simulink model "rect_design"  (R2016a)
settings: Solver=ode4  StartTime=0.0  StopTime=0.5  FixedStep=1e-5  RelTol=1e-3
undefined symbols (not defined in the file or in its folder): Lload
libraries: powerlib x12, powerlib_meascontrol x5, simulink x4
settings Model: Creator=ugurm  LastModifiedBy=mesutto
settings DataIOCC: LimitDataPoints=on  SaveFormat=Array
settings DebuggingCC: UnderspecifiedInitializationDetection=Classic  MergeDetectMultiDrivingBlocksExec=none  SolverPrmCheckMsg=warning  UnconnectedInputMsg=none  UnconnectedOutputMsg=none  UnconnectedLineMsg=none  StateNameClashWarn=warning
settings HardwareCC: ProdBitPerPointer=32  ProdLargestAtomicFloat=None  ProdIntDivRoundTo=Undefined  ProdEndianess=Unspecified  ProdWordSize=32  ProdHWDeviceType=32-bit Generic
settings ModelReferenceCC: PropagateSignalLabelsOutOfModel=off
settings ConfigComp: CovModelRefEnable=Off

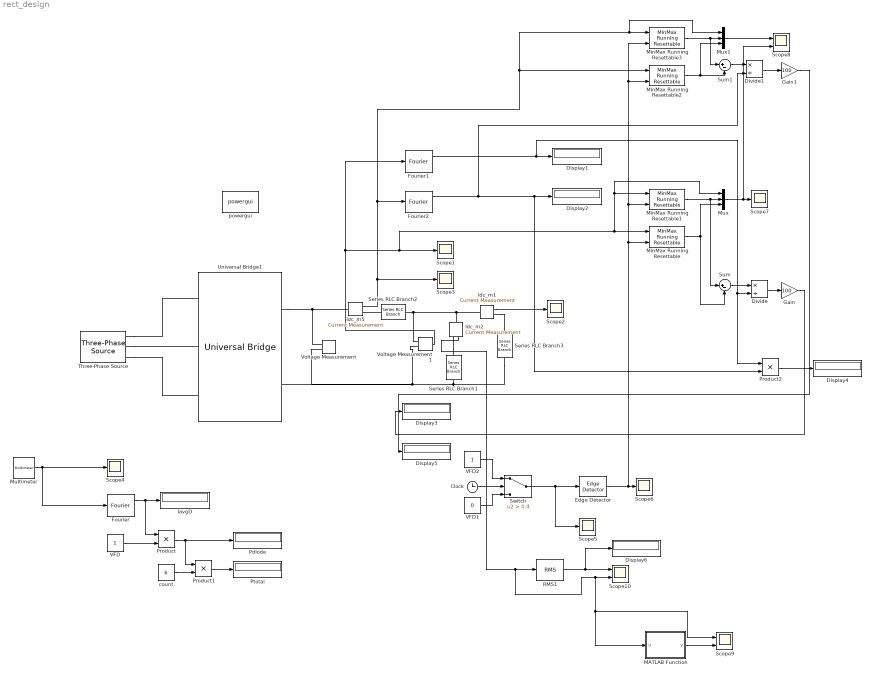
== system rect_design ==
  Clock : Clock
  Display{1..6} (6 alike) : Display
  Divide : Product  Inputs=*/
  Divide1 : Product  Inputs=*/
  Edge Detector : powerlib_meascontrol/Logic/Edge Detector  model=Rising  ic=0  Ts=0
  Fourier : powerlib_meascontrol/Measurements/Fourier  Freq=50  n=0  InInit=[0, 0]  Ts=0
  Fourier1 : powerlib_meascontrol/Measurements/Fourier  Freq=50  n=0  InInit=[0, 0]  Ts=0
  Fourier2 : powerlib_meascontrol/Measurements/Fourier  Freq=50  n=0  InInit=[0, 0]  Ts=0
  Gain : Gain  Gain=100
  Gain1 : Gain  Gain=100
  IavgD : Display
  Idc_m1 : powerlib/Measurements/Current Measurement  PhasorSimulation=off  OutputType=Complex  PSBequivalent=0
  Idc_m2 : powerlib/Measurements/Current Measurement  PhasorSimulation=off  OutputType=Complex  PSBequivalent=0
  Idc_m5 : powerlib/Measurements/Current Measurement  PhasorSimulation=off  OutputType=Complex  PSBequivalent=0
  MATLAB Function : MATLAB Function  TreatAsAtomicUnit=on
  MinMax Running Resettable : simulink/Math Operations/MinMax Running Resettable  Function=min  vinit=1000
  MinMax Running Resettable1 : simulink/Math Operations/MinMax Running Resettable  Function=max  vinit=0
  MinMax Running Resettable2 : simulink/Math Operations/MinMax Running Resettable  Function=min  vinit=1000
  MinMax Running Resettable3 : simulink/Math Operations/MinMax Running Resettable  Function=max  vinit=0
  Multimeter : powerlib/Measurements/Multimeter  PhasorSimulation=off  OutputType=Complex  sel=1  L=6  Gain=1  yselected={'Isw1: Universal Bridge1'};  PSBOutputType=1  PSBequivalent=0  AxesSetting=[0,0.1,-100,100]  Display=0  SavedBlockNames=-11
  Mux : Mux  Inputs=3
  Mux1 : Mux  Inputs=3
  Pdiode : Display
  Product : Product
  Product1 : Product
  Product2 : Product
  Ptotal : Display
  RMS1 : powerlib_meascontrol/Measurements/RMS  TrueRMS=on  Freq=50  RMSInit=120  Ts=0
  Scope{1..7} (7 alike) : Scope
  Scope10 : Scope  NumInputPorts=2
  Scope8 : Scope  NumInputPorts=2
  Scope9 : Scope  NumInputPorts=2
  Series RLC Branch1 : powerlib/Elements/Series RLC Branch  LConnTagsString=__new0  RConnTagsString=__new0  BranchType=C  Resistance=30  Inductance=Lload  SetiL0=off  InitialCurrent=0  Capacitance=1.2e-3  Setx0=off  InitialVoltage=0  Measurements=None
  Series RLC Branch2 : powerlib/Elements/Series RLC Branch  LConnTagsString=__new0  RConnTagsString=__new0  BranchType=RL  Resistance=1e-3  Inductance=3e-3  SetiL0=off  InitialCurrent=0  Capacitance=10e-3  Setx0=off  InitialVoltage=0  Measurements=None
  Series RLC Branch3 : powerlib/Elements/Series RLC Branch  LConnTagsString=__new0  RConnTagsString=__new0  BranchType=R  Resistance=30  Inductance=Lload  SetiL0=off  InitialCurrent=0  Capacitance=1e-6  Setx0=off  InitialVoltage=0  Measurements=None
  Sum : Sum  Inputs=|+-
  Sum1 : Sum  Inputs=|+-
  Switch : Switch  Criteria=u2 > Threshold  Threshold=0.4
  Three-Phase Source : powerlib/Electrical Sources/Three-Phase Source  InternalConnection=Yg  VoltagePhases=off  Voltage=400  PhaseAngle=0  Voltage_phases=[25e3 25e3 25e3]/sqrt(3)  PhaseAngles_phases=[0 -120 +120]  Frequency=50  NonIdealSource=off  SpecifyImpedance=off  Resistance=0.8929  Inductance=16.58e-3  ShortCircuitLevel=100e6  BaseVoltage=25e3  XRratio=7  BusType=swing  Pref=10e3  Qref=0  Prefabc=[10e3, 10e3, 10e3]  Qrefabc=[0, 0, 0]  Qmin=-inf  Qmax=inf
  Universal Bridge1 : powerlib/Power Electronics/Universal Bridge  Arms=3  SnubberResistance=1e5  SnubberCapacitance=inf  Device=Diodes  Ron=1e-6  Lon=0  ForwardVoltages="[  0  0  ]"  ForwardVoltage=0  GTOparameters=[ 10e-6 , 20e-6 ]  IGBTparameters=[0,0]  Measurements=Device currents  Measurements_2=None  converterType=Rectifier
  VFD : Constant
  VFD1 : Constant  Value=0
  VFD2 : Constant
  Voltage Measurement : powerlib/Measurements/Voltage Measurement  PhasorSimulation=off  OutputType=Complex  PSBequivalent=0
  Voltage Measurement1 : powerlib/Measurements/Voltage Measurement  PhasorSimulation=off  OutputType=Complex  PSBequivalent=0
  count : Constant  Value=6
  powergui : powerlib/powergui  Priority=1  SimulationMode=Discrete  SolverType=Tustin  SampleTime=1e-5  frequency=60  SPID=off  DisableSnubberDevices=off  DisableRonSwitches=off  DisableVfSwitches=off  SwTol=0  DisplayEquations=off  Interpol=off  ExternalGateDelay=off  methode=off  Ts=0  FunctionMessages=off  echomessages=off  HookPort=off  EnableUseOfTLC=off  x0status=blocks  frequencyindice=0  Pbase=100e6  ErrMax=1e-4  Iterations=50  UnitsV=kV  UnitsW=MW  buscounter=0  RestoreLinks=warning  ResistiveCurrentMeasurement=off  Frange=[0:2:500]  Ylog=off  Xlog=on  ShowGrid=off  save=off  variable=ZData  structure=Vdc  ZoomFFT=off  StartTime=0.04  cycles=5  DisplayStyle=5  fundamental=50  FreqAxis=off  MaxFrequency=30000  frequencyindicesteady=1  RmsSteady=1  display=off
  wires:
  Idc_m1/1 -> Scope2/1
  Multimeter/1 -> Scope4/1, Fourier/1
  Fourier/1 -> Product/1, IavgD/1
  Voltage Measurement1/1 -> Fourier1/1, MinMax Running Resettable1/1, Mux/1, MinMax Running Resettable/1, Scope1/1
  VFD/1 -> Product/2
  Product/1 -> Product1/1, Pdiode/1
  count/1 -> Product1/2
  Product1/1 -> Ptotal/1
  Idc_m5/1 -> Mux1/1, MinMax Running Resettable3/1, MinMax Running Resettable2/1, Fourier2/1, Scope3/1
  Clock/1 -> Switch/2
  VFD1/1 -> Switch/3
  VFD2/1 -> Switch/1
  Switch/1 -> Edge Detector/1, Scope5/1
  Edge Detector/1 -> MinMax Running Resettable/2, MinMax Running Resettable3/2, MinMax Running Resettable2/2, MinMax Running Resettable1/2, Scope6/1
  MinMax Running Resettable/1 -> Mux/3, Sum/2
  MinMax Running Resettable1/1 -> Mux/2, Sum/1
  Mux/1 -> Scope8/2, Scope7/1
  Sum/1 -> Divide/1
  Divide/1 -> Gain/1
  Gain/1 -> Display3/1
  Product2/1 -> Display4/1
  Fourier1/1 -> Product2/1, Divide/2, Display1/1
  MinMax Running Resettable2/1 -> Mux1/3, Sum1/2
  MinMax Running Resettable3/1 -> Mux1/2, Sum1/1
  Mux1/1 -> Scope8/1
  Sum1/1 -> Divide1/1
  Divide1/1 -> Gain1/1
  Gain1/1 -> Display5/1
  Fourier2/1 -> Divide1/2, Product2/2, Display2/1
  Idc_m2/1 -> RMS1/1, Scope9/1, MATLAB Function/1(u), Scope10/2
  RMS1/1 -> Scope10/1, Display6/1
  MATLAB Function/1(y) -> Scope9/2
  connections:
  Universal Bridge1/RConn1 -- Voltage Measurement/LConn1 -- Idc_m5/LConn1
  Series RLC Branch1/RConn1 -- Universal Bridge1/RConn2 -- Voltage Measurement/LConn2 -- Voltage Measurement1/LConn2 -- Series RLC Branch3/RConn1
  Idc_m1/RConn1 -- Series RLC Branch3/LConn1
  Three-Phase Source/RConn1 -- Universal Bridge1/LConn1
  Three-Phase Source/RConn2 -- Universal Bridge1/LConn2
  Three-Phase Source/RConn3 -- Universal Bridge1/LConn3
  Series RLC Branch2/RConn1 -- Idc_m5/RConn1
  Series RLC Branch1/LConn1 -- Idc_m2/RConn1
  Series RLC Branch2/LConn1 -- Voltage Measurement1/LConn1 -- Idc_m1/LConn1 -- Idc_m2/LConn1

== matlab function rect_design/MATLAB Function ==
  data: u input; y output
function y = fcn(u)
%#codegen

y = 2*u;
